simulink subsystem "clock_and_data_recovery"  (R2022b)
settings: Solver=VariableStepAuto  StartTime=0.0  StopTime=10.0  RelTol=1e-3
settings Model: Creator=Ali-Laptop  LastModifiedBy=Ali-Laptop

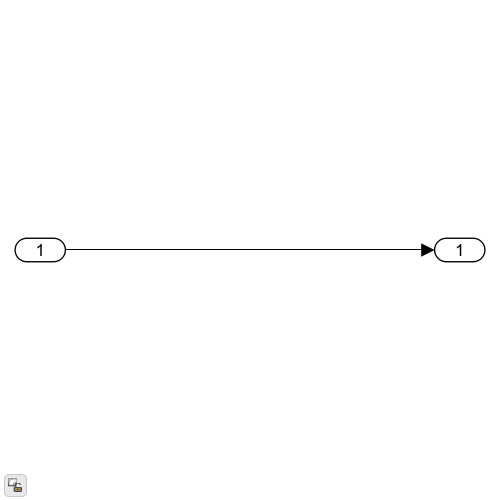
[thumbnail: Simulink's stored preview of the top-level diagram]
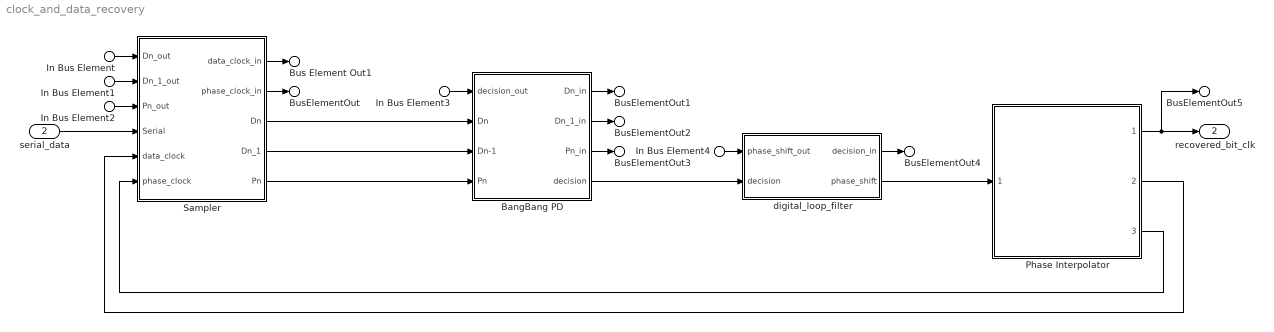
== system clock_and_data_recovery ==
  In Bus Element : Inport  PortName=digital_out  Element=Dn_out
  In Bus Element1 : Inport  PortName=digital_out  Element=Dn_1_out
  In Bus Element2 : Inport  PortName=digital_out  Element=Pn_out
  In Bus Element3 : Inport  PortName=digital_out  Element=decision_out
  In Bus Element4 : Inport  PortName=digital_out  Element=phase_shift
  serial_data : Inport  Port=2
  BangBang PD : Subsystem
  Phase Interpolator : Subsystem  ReferencedSubsystem=phase_interpolator
  Sampler : Subsystem
  digital_loop_filter : Subsystem
  Bus Element Out1 : Outport  PortName=digital_in  Element=data_clock
  BusElementOut : Outport  PortName=digital_in  Element=phase_clock
  BusElementOut1 : Outport  PortName=digital_in  Element=Dn
  BusElementOut2 : Outport  PortName=digital_in  Element=Dn_1
  BusElementOut3 : Outport  PortName=digital_in  Element=Pn
  BusElementOut4 : Outport  PortName=digital_in  Element=Decision
  BusElementOut5 : Outport  PortName=digital_in  Element=recovered_clock
  recovered_bit_clk : Outport  Port=2
  wires:
  Phase Interpolator/1 -> BusElementOut5/1, recovered_bit_clk/1
  Sampler/1(data_clock_in) -> Bus Element Out1/1
  Sampler/2(phase_clock_in) -> BusElementOut/1
  BangBang PD/1(Dn_in) -> BusElementOut1/1
  BangBang PD/2(Dn_1_in) -> BusElementOut2/1
  BangBang PD/3(Pn_in) -> BusElementOut3/1
  digital_loop_filter/1(decision_in) -> BusElementOut4/1
  In Bus Element/1 -> Sampler/1(Dn_out)
  In Bus Element1/1 -> Sampler/2(Dn_1_out)
  In Bus Element2/1 -> Sampler/3(Pn_out)
  In Bus Element3/1 -> BangBang PD/1(decision_out)
  In Bus Element4/1 -> digital_loop_filter/1(phase_shift_out)
  Sampler/5(Pn) -> BangBang PD/4(Pn)
  Sampler/4(Dn_1) -> BangBang PD/3(Dn-1)
  Sampler/3(Dn) -> BangBang PD/2(Dn)
  serial_data/1 -> Sampler/4(Serial)
  Phase Interpolator/3 -> Sampler/6(phase_clock)
  Phase Interpolator/2 -> Sampler/5(data_clock)
  digital_loop_filter/2(phase_shift) -> Phase Interpolator/1
  BangBang PD/4(decision) -> digital_loop_filter/2(decision)

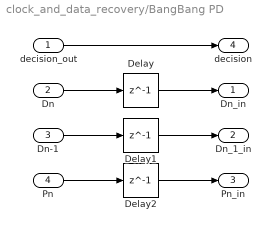
== system clock_and_data_recovery/BangBang PD ==
  decision_out : Inport
  Dn : Inport  Port=2
  Dn-1 : Inport  Port=3
  Pn : Inport  Port=4
  Delay : Delay  DelayLength=1
  Delay1 : Delay  DelayLength=1
  Delay2 : Delay  DelayLength=1
  Dn_in : Outport
  Dn_1_in : Outport  Port=2
  Pn_in : Outport  Port=3
  decision : Outport  Port=4
  wires:
  Delay2/1 -> Pn_in/1
  Delay1/1 -> Dn_1_in/1
  Delay/1 -> Dn_in/1
  Dn/1 -> Delay/1
  Dn-1/1 -> Delay1/1
  Pn/1 -> Delay2/1
  decision_out/1 -> decision/1

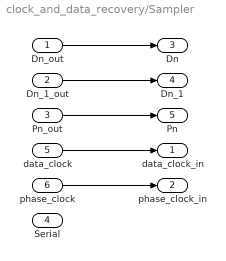
== system clock_and_data_recovery/Sampler ==
  Dn_out : Inport
  Dn_1_out : Inport  Port=2
  Pn_out : Inport  Port=3
  Serial : Inport  Port=4
  data_clock : Inport  Port=5
  phase_clock : Inport  Port=6
  data_clock_in : Outport
  phase_clock_in : Outport  Port=2
  Dn : Outport  Port=3
  Dn_1 : Outport  Port=4
  Pn : Outport  Port=5
  wires:
  phase_clock/1 -> phase_clock_in/1
  data_clock/1 -> data_clock_in/1
  Pn_out/1 -> Pn/1
  Dn_1_out/1 -> Dn_1/1
  Dn_out/1 -> Dn/1

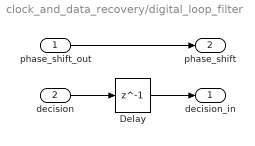
== system clock_and_data_recovery/digital_loop_filter ==
  phase_shift_out : Inport
  decision : Inport  Port=2
  Delay : Delay  DelayLength=1
  decision_in : Outport
  phase_shift : Outport  Port=2
  wires:
  Delay/1 -> decision_in/1
  phase_shift_out/1 -> phase_shift/1
  decision/1 -> Delay/1
